simulink model "EXP_03_MPPT"  (R2025a)
settings: Solver=VariableStepAuto  StartTime=0.0  StopTime=2  RelTol=1e-3
libraries: spsSeriesRLCBranchLib x4, spsDiodeLib x2, spsCurrentMeasurementLib x1, spsMosfetLib x1, spsPWMGeneratorDCDCLib x1, spsPVArrayLib x1, spsVoltageMeasurementLib x1, sps_lib x1
settings Model: Creator=praga  LastModifiedBy=praga

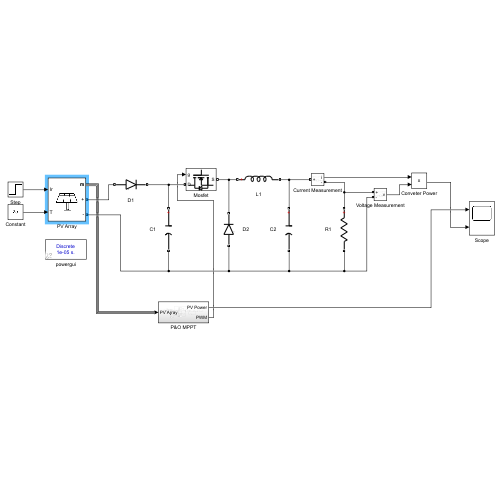
[thumbnail: Simulink's stored preview of the top-level diagram]
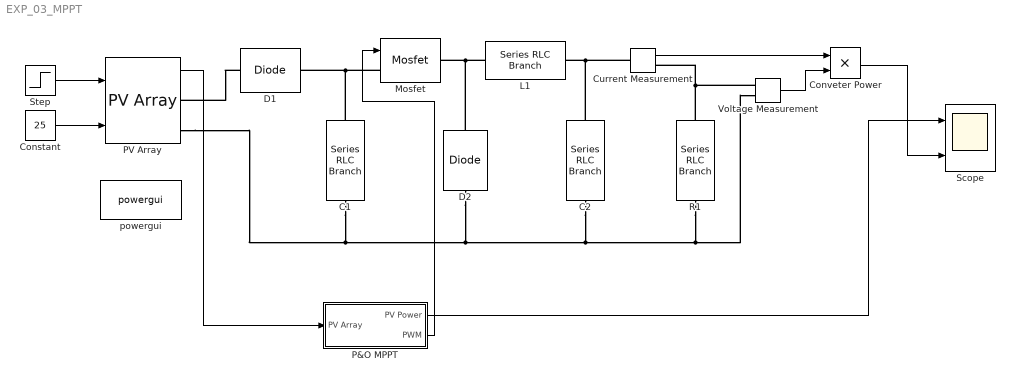
== system EXP_03_MPPT ==
  C1 : spsSeriesRLCBranchLib/Series RLC Branch  LConnTagsString=__new0  RConnTagsString=__new0  BranchType=C  Resistance=1  Inductance=1e-3  SetiL0=off  InitialCurrent=0  Capacitance=50e-6  Setx0=off  InitialVoltage=0  Measurements=None
  C2 : spsSeriesRLCBranchLib/Series RLC Branch  LConnTagsString=__new0  RConnTagsString=__new0  BranchType=C  Resistance=1  Inductance=1e-3  SetiL0=off  InitialCurrent=0  Capacitance=50e-6  Setx0=off  InitialVoltage=0  Measurements=None
  Constant : Constant  Value=25
  Conveter Power : Product
  Current Measurement : spsCurrentMeasurementLib/Current Measurement  PhasorSimulation=off  OutputType=Complex  PSBequivalent=0
  D1 : spsDiodeLib/Diode  Ron=0.001  Lon=0  Vf=0.8  IC=0  UseSnubber=0  Rs=0  Cs=0  Measurements=off
  D2 : spsDiodeLib/Diode  Ron=0.001  Lon=0  Vf=0.8  IC=0  UseSnubber=0  Rs=0  Cs=0  Measurements=off
  L1 : spsSeriesRLCBranchLib/Series RLC Branch  LConnTagsString=__new0  RConnTagsString=__new0  BranchType=L  Resistance=1  Inductance=1e-3  SetiL0=off  InitialCurrent=0  Capacitance=1e-6  Setx0=off  InitialVoltage=0  Measurements=None
  Mosfet : spsMosfetLib/Mosfet  Ron=0.1  Lon=0  Rd=0.01  Vfd=0  IC=0  Rs=1e5  Cs=inf  Measurements=off
  P&O MPPT : Subsystem
  PV Array : spsPVArrayLib/PV Array  Npar=40  Nser=10  PlotType=array @ 1000 W/m2 & specified temperatures  S_vec="[ 1000  500  100 ]"  Temp_C_vec="[ 45 25  ]"  ModuleName=User-defined  PlotWhenSelected=off  Pm=213.15  Ncell=60  Voc=36.3  Isc=7.84  Vm=29  Im=7.35  beta_Voc_pc=-0.36099  alpha_Isc_pc=0.102  beta_Voc=-0.13104  alpha_Isc=0.0079968  IL=7.8654  I0=2.9273e-10  nI=0.98119  Rsh=313.0553  Rs=0.39381  RobustModel=off  RobustCellTemperature=313.3991  BAL=on  Tc=1e-6  Tfilter=5e-5
  R1 : spsSeriesRLCBranchLib/Series RLC Branch  LConnTagsString=__new0  RConnTagsString=__new0  BranchType=R  Resistance=1000  Inductance=0  SetiL0=off  InitialCurrent=0  Capacitance=0  Setx0=off  InitialVoltage=0  Measurements=None
  Scope : Scope  NumInputPorts=2
      settings: Title=Converter Power  ActiveDisplayYMinimum=-7.971965290253535  ActiveDisplayYMaximum=71.747687612281837  YLabel=Power (W)
  Step : Step  SampleTime=0
  Voltage Measurement : spsVoltageMeasurementLib/Voltage Measurement  PhasorSimulation=off  OutputType=Complex  PSBequivalent=0
  powergui : sps_lib/powergui  Priority=1  SimulationMode=Discrete  SampleTime=1e-05  frequency=60  Iterations=50  frequencyindice=0  Pbase=100e6  ErrMax=1e-4  UnitsV=kV  UnitsW=MW  buscounter=0  FunctionMessages=off  echomessages=off  EnableUseOfTLC=off  CurrentSourceSwitches=off  DisableSnubberDevices=off  DisableRonSwitches=off  DisableVfSwitches=off  DisplayEquations=off  AutomaticDiscreteSolvers=off  SolverType=Tustin/Backward Euler (TBE)  Interpol=off  ExternalGateDelay=off  methode=off  Ts=100  x0status=blocks  SPID=on  SwTol=0  HookPort=off  NonlinearTolerance=1e-4  nMaxIteration=100  ContinueOnMaxIteration=off  RestoreLinks=warning  ResistiveCurrentMeasurement=off  Frange=[0:2:500]  Ylog=off  Xlog=on  ShowGrid=off  save=off  variable=ZData  structure=0  ZoomFFT=off  StartTime=0.0  cycles=1  DisplayStyle=1  fundamental=60  FreqAxis=off  MaxFrequency=1000  frequencyindicesteady=1  RmsSteady=1  display=off
  wires:
  PV Array/1 -> P&O MPPT/1(PV Array)
  Current Measurement/1 -> Conveter Power/1
  Voltage Measurement/1 -> Conveter Power/2
  P&O MPPT/1(PV Power) -> Scope/1
  P&O MPPT/2(PWM) -> Mosfet/1
  Constant/1 -> PV Array/2
  Step/1 -> PV Array/1
  Conveter Power/1 -> Scope/2
  connections:
  D1/LConn1 -- PV Array/RConn1
  Mosfet/LConn1 -- D1/RConn1 -- C1/LConn1
  L1/LConn1 -- D2/RConn1 -- Mosfet/RConn1
  Current Measurement/LConn1 -- C2/LConn1 -- L1/RConn1
  Voltage Measurement/LConn1 -- Current Measurement/RConn1 -- R1/LConn1
  PV Array/RConn2 -- C1/RConn1 -- D2/LConn1 -- C2/RConn1 -- R1/RConn1 -- Voltage Measurement/LConn2

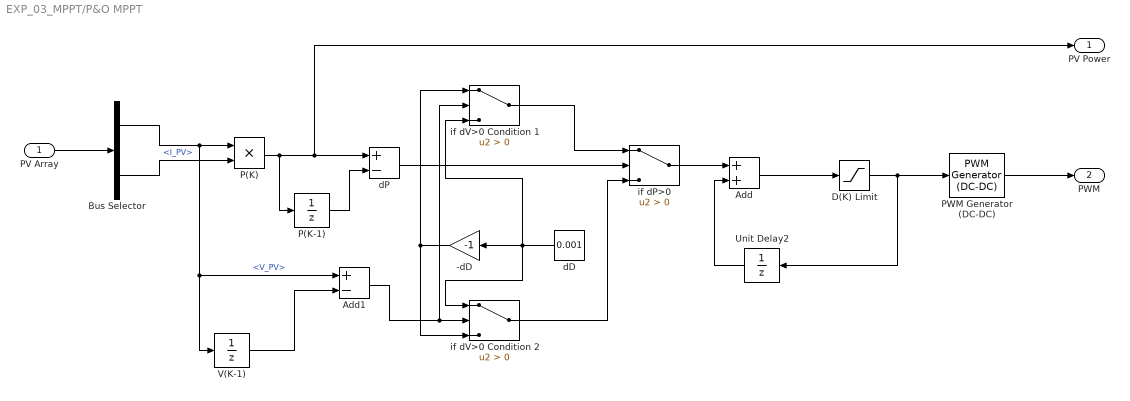
== system EXP_03_MPPT/P&O MPPT ==
  PV Array : Inport
  -dD : Gain  Gain=-1
  Add : Sum
  Add1 : Sum  Inputs=+-
  Bus Selector : BusSelector  OutputSignals=V_PV,I_PV
  D(K) Limit : Saturate  UpperLimit=1  LowerLimit=0
  P(K) : Product
  P(K-1) : UnitDelay  SampleTime=1e-5  HasFrameUpgradeWarning=on
  PWM Generator (DC-DC) : spsPWMGeneratorDCDCLib/PWM Generator (DC-DC)  Fsw=5000  Ts=0
  Unit Delay2 : UnitDelay  SampleTime=-1  HasFrameUpgradeWarning=on
  V(K-1) : UnitDelay  SampleTime=1e-5  HasFrameUpgradeWarning=on
  dD : Constant  Value=0.001
  dP : Sum  Inputs=+-
  if dP>0 : Switch  Criteria=u2 > Threshold  SaturateOnIntegerOverflow=off  InputSameDT=off
  if dV>0 Condition 1 : Switch  Criteria=u2 > Threshold  SaturateOnIntegerOverflow=off  InputSameDT=off
  if dV>0 Condition 2 : Switch  Criteria=u2 > Threshold  SaturateOnIntegerOverflow=off  InputSameDT=off
  PV Power : Outport
  PWM : Outport  Port=2
  wires:
  PV Array/1 -> Bus Selector/1
  Bus Selector/2 -> P(K)/2  "<I_PV>"
  Bus Selector/1 -> V(K-1)/1, Add1/1, P(K)/1  "<V_PV>"
  P(K)/1 -> P(K-1)/1, dP/1, PV Power/1
  P(K-1)/1 -> dP/2
  V(K-1)/1 -> Add1/2
  dD/1 -> if dV>0 Condition 1/3, if dV>0 Condition 2/1, -dD/1
  if dV>0 Condition 1/1 -> if dP>0/1
  Add1/1 -> if dV>0 Condition 2/2, if dV>0 Condition 1/2
  if dV>0 Condition 2/1 -> if dP>0/3
  -dD/1 -> if dV>0 Condition 1/1, if dV>0 Condition 2/3
  dP/1 -> if dP>0/2
  if dP>0/1 -> Add/1
  Unit Delay2/1 -> Add/2
  Add/1 -> D(K) Limit/1
  D(K) Limit/1 -> Unit Delay2/1, PWM Generator (DC-DC)/1
  PWM Generator (DC-DC)/1 -> PWM/1
